simulink model "TrafficLights"  (R2019b)
settings: Solver=VariableStepAuto  StartTime=0.0  StopTime=100  RelTol=1e-3
settings Model: Creator=ip  LastModifiedBy=ip

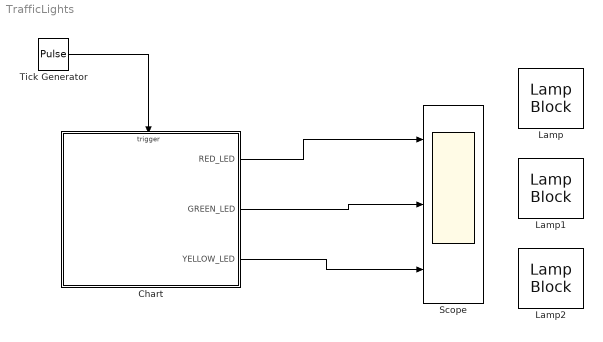
== system TrafficLights ==
  Chart : Stateflow chart  BlockKeywords=__PRM__SERIALIZED__DATA__:Stateflow Chart,Stateflow Diagram  TreatAsAtomicUnit=on
  Lamp : LampBlock
  Lamp1 : LampBlock
  Lamp2 : LampBlock
  Scope : Scope  NumInputPorts=3
  Tick Generator : DiscretePulseGenerator  PulseType=Time based  Period=0.04  PulseWidth=50
  wires:
  Tick Generator/1 -> Chart/Trigger
  Chart/2(GREEN_LED) -> Scope/2
  Chart/1(RED_LED) -> Scope/1
  Chart/3(YELLOW_LED) -> Scope/3

== stateflow chart TrafficLights/Chart ==
  state Stop
    entry: RED_LED = 1;
    exit: RED_LED = 0;
  state Go
    entry: GREEN_LED = 1;
    exit: GREEN_LED = 0;
  state PrepareToStop
    entry: YELLOW_LED = 1;
    exit: YELLOW_LED = 0;
  (default) -> Stop
  PrepareToStop -> Stop : after(10,sec)
  Stop -> Go : after(30,sec)
  Go -> PrepareToStop : after(20,sec)
  data: RED_LED output uint8; GREEN_LED output uint8; YELLOW_LED output uint8
  events: tick input RISING_EDGE_EVENT
